simulink model "fifo3"  (R2025a)
settings: Solver=VariableStepAuto  StartTime=0.0  StopTime=10.0  RelTol=1e-3
libraries: StdLib x10, PaperLib x3
settings Model: Creator=david  LastModifiedBy=peter
settings OptimizationCC: ReuseModelBlockBuffer=off
settings RTWCC: GPUComputeCapability=3.5

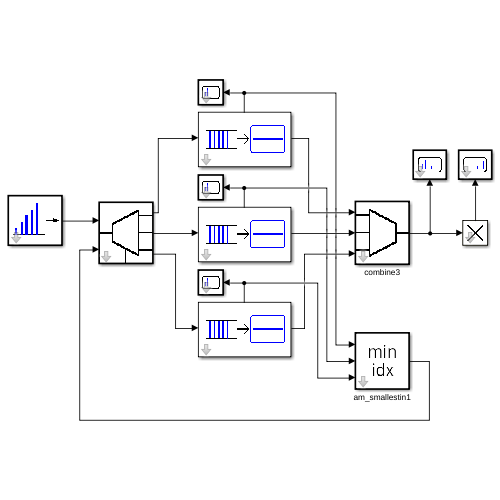
[thumbnail: Simulink's stored preview of the top-level diagram]
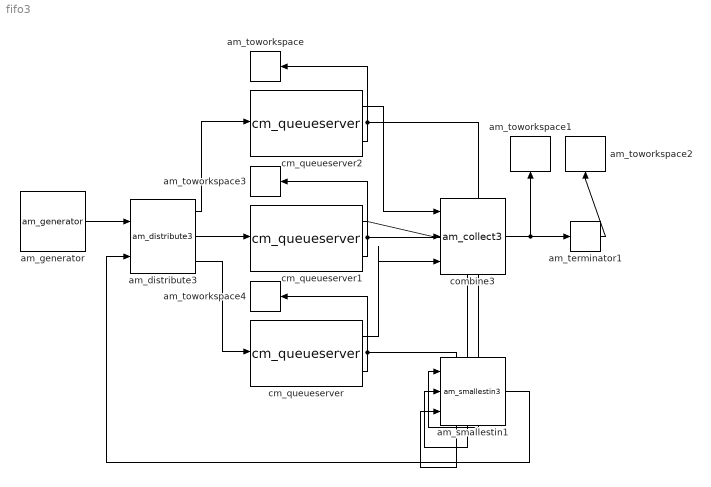
== system fifo3 ==
  am_distribute3 : StdLib/am_distribute3  port0=1  field="\"\""  tau=[0,1]  debug=0
      settings: SourceProductName=Routing
  am_generator : StdLib/am_generator  tG=1  n0=1  nG=13  tD=[0,2]  debug=0
      settings: SourceProductName=Sources
  am_smallestin1 : StdLib/am_smallestin3  val0=0  tau=[0,1]  debug=0
      settings: SourceProductName=Routing
  am_terminator1 : StdLib/am_terminator  tau=[0,1]  debug=0
  am_toworkspace : StdLib/am_toworkspace  varname="\"nqs1\""  t0=0  format="\"vector\""  tau=[0,5]  debug=0
  am_toworkspace1 : StdLib/am_toworkspace  varname="\"output\""  t0=0  format="\"vector\""  tau=[0,5]  debug=0
  am_toworkspace2 : StdLib/am_toworkspace  varname="\"thrput\""  t0=0  format="\"vector\""  tau=[0,5]  debug=0
  am_toworkspace3 : StdLib/am_toworkspace  varname="\"nqs2\""  t0=0  format="\"vector\""  tau=[0,5]  debug=0
  am_toworkspace4 : StdLib/am_toworkspace  varname="\"nqs3\""  t0=0  format="\"vector\""  tau=[0,5]  debug=0
  cm_queueserver : PaperLib/cm_queueserver  ts=4.5  tau=[0,1]  debug=0
      link override am_toworkspace: varname="\"nq3\""
  cm_queueserver1 : PaperLib/cm_queueserver  ts=4.5  tau=[0,1]  debug=0
      link override am_toworkspace: varname="\"nq2\""
  cm_queueserver2 : PaperLib/cm_queueserver  ts=4.5  tau=[0,1]  debug=0
  combine3 : StdLib/am_collect3  tD=[0,2]  tau=[0,1]  debug=0
      settings: SourceProductName=Routing
  wires:
  am_distribute3/1 -> cm_queueserver2/1
  am_distribute3/2 -> cm_queueserver1/1
  am_distribute3/3 -> cm_queueserver/1
  cm_queueserver1/1 -> combine3/2
  cm_queueserver2/1 -> combine3/1
  cm_queueserver/1 -> combine3/3
  cm_queueserver2/2 -> am_toworkspace/1, am_smallestin1/1
  cm_queueserver1/2 -> am_toworkspace3/1, am_smallestin1/2
  cm_queueserver/2 -> am_toworkspace4/1, am_smallestin1/3
  am_smallestin1/1 -> am_distribute3/2
  am_generator/1 -> am_distribute3/1
  combine3/1 -> am_toworkspace1/1, am_terminator1/1
  am_terminator1/1 -> am_toworkspace2/1
